simulink model "If_Then_Else_2018a"  (R2018a)
settings: Solver=VariableStepAuto  StartTime=0.0  StopTime=10.0  RelTol=1e-3
settings Model: Creator=apple  LastModifiedBy=apple
settings DataIOCC: ReturnWorkspaceOutputs=on
settings SFSimCC: SimUseLocalCustomCode=on
settings RTWCC: RTWUseLocalCustomCode=on

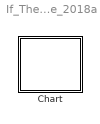
== system If_Then_Else_2018a ==
  Chart : Stateflow chart  TreatAsAtomicUnit=on

== stateflow chart If_Then_Else_2018a/Chart ==
  state C
    en:fprintf("Entry C");
    du:fprintf("During C");
    ex:fprintf("Exit C");
  state A
    en:fprintf("Entry A");
    du:fprintf("During A");
    ex:fprintf("Exit A");
  state B
    en:fprintf("Entry B");
    du:fprintf("During B");
    ex:fprintf("Exit B");
  state D
    en:fprintf("Entry D");
    du:fprintf("During D");
    ex:fprintf("Exit D");
  (junction 9) -> C [order 1] : [x> 0]{fprintf("Condition Action2");}
  (default) -> A : {x = 0;}
  A -> (junction 9) : E_one/{fprintf("Transition Action1");}
  (junction 9) -> B [order 2] : [x> -1]{fprintf("Condition Action3");}
  (junction 9) -> D [order 3]
